simulink model "ExampleQueryChassis"  (Simulink 9.2)
settings: Solver=FixedStepDiscrete  StartTime=0.0  StopTime=inf  FixedStep=0.001  RelTol=1e-3  EnableMultiTasking=on
libraries: rFproPhysicsLib x2
settings Model: Creator=marine  LastModifiedBy=SeanKavanagh
settings OptimizationCC: ExpressionDepthLimit=2147483647  InitFltsAndDblsToZero=on
settings DebuggingCC: SaveWithParameterizedLinksMsg=none  SolverPrmCheckMsg=warning
settings HardwareCC: TargetBitPerPointer=64  TargetBitPerSizeT=64  TargetBitPerPtrDiffT=64  TargetLongLongMode=on  TargetIntDivRoundTo=Zero  TargetEndianess=LittleEndian  TargetWordSize=64  TargetHWDeviceType=MATLAB Host  ProdEqTarget=off
settings RTWCC: SystemTargetFile=rsim.tlc  TemplateMakefile=rsim_default_tmf  Description=Rapid Simulation Target  TargetLang=C++
settings RSimTargetCC: PreserveStateflowLocalDataDimensions=off

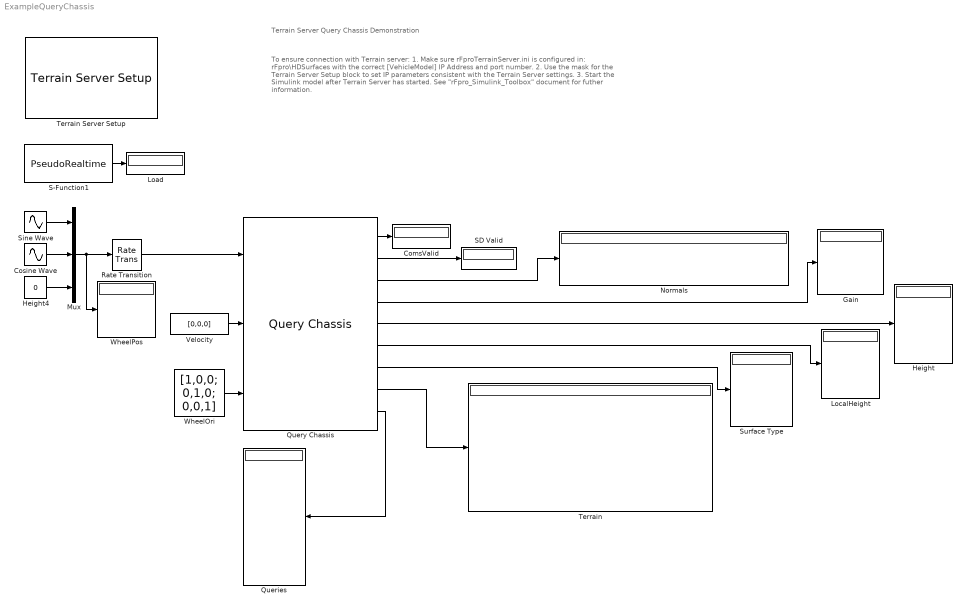
== system ExampleQueryChassis ==
  note: Terrain Server Query Chassis Demonstration
  note: To ensure connection with Terrain server:
      |
      | 1. Make sure rFproTerrainServer.ini is configured in: rFpro\HDSurfaces with the correct
      |     [VehicleModel] IP Address and port number.
      |
      | 2. Use the mask for the Terrain Server Setup block to set IP parameters consistent with
      |     the Terrain Server settings.
      |
      | 3. Start the Simulink model after Terrain Server has started.
      |
      | See "rFpro_Simulink_Toolbox" document for futher information.
  ComsValid : Display
  Cosine Wave : Sin  Amplitude=60  Bias=-620  Frequency=20*pi/20  Phase=pi/2  SampleTime=0.001
  Gain : Display
  Height : Display
  Height4 : Constant  Value=0
  Load : Display
  LocalHeight : Display
  Mux : Mux  Inputs=3
  Normals : Display
  Queries : Display
  Query Chassis : rFproPhysicsLib/Terrain Server Blocks/Query Chassis  points=[0,0,0; 0,0,1; 1,2,-1; 4,5,5.1]  NumChassisPts=0  iso_mode=on  sampletime=0.001  phase_delay=0  roundtrip_frames=2  queryID_start=1  queryID_step=1  useReverseByteOrder=off  rFpro__TS_platform=Remote Model - Default
  Rate Transition : RateTransition
  S-Function1 : S-Function  FunctionName=PseudoRealtime  Parameters=0.001  SFunctionDeploymentMode=off  EnableBusSupport=off
  SD Valid : Display
  Sine Wave : Sin  Amplitude=60  Bias=821.6  Frequency=2*pi/20  SampleTime=0.001
  Surface Type : Display
  Terrain : Display
  Terrain Server Setup : rFproPhysicsLib/Terrain Server Blocks/Terrain Server Setup  Priority=0  track_name=''  tyre_config=[]  points_config=[]  iso=on  triggerOnHeartbeat=off  heartbeat_latency=1750  rFpro__platform=Remote Model - Default  ts_address='127.0.0.1'  ts_port=11006  sendSampleTime=-1  sl_address='127.0.0.1'  sl_port=11002  receiveSampleTime=-1  maxUDPMsgs=2  useReverseByteOrder=off
  Velocity : Constant  Value=[0,0,0]
  WheelOri : Constant  Value=[1,0,0; 0,1,0; 0,0,1]
  WheelPos : Display
  wires:
  S-Function1/1 -> Load/1
  Sine Wave/1 -> Mux/1
  Cosine Wave/1 -> Mux/2
  Height4/1 -> Mux/3
  Mux/1 -> WheelPos/1, Rate Transition/1
  Query Chassis/1 -> ComsValid/1
  Query Chassis/2 -> SD Valid/1
  Query Chassis/4 -> Gain/1
  Query Chassis/5 -> Height/1
  Query Chassis/6 -> LocalHeight/1
  Query Chassis/7 -> Surface Type/1
  WheelOri/1 -> Query Chassis/3
  Velocity/1 -> Query Chassis/2
  Rate Transition/1 -> Query Chassis/1
  Query Chassis/9 -> Queries/1
  Query Chassis/8 -> Terrain/1
  Query Chassis/3 -> Normals/1
